simulink subsystem "Log"  (R2024b)
settings: Solver=VariableStepAuto  StartTime=0.0  StopTime=10.0  RelTol=1e-3
settings Model: Creator=Tong  LastModifiedBy=Tong

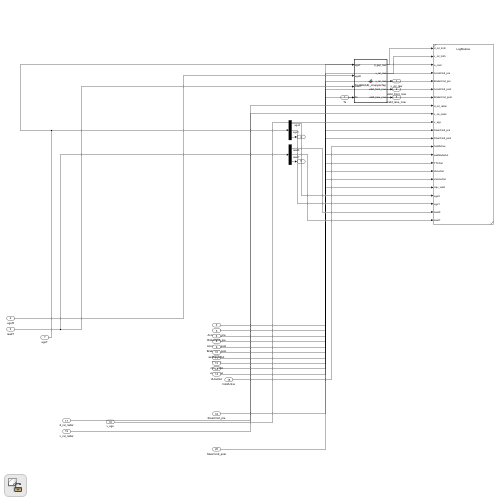
[thumbnail: Simulink's stored preview of the top-level diagram]
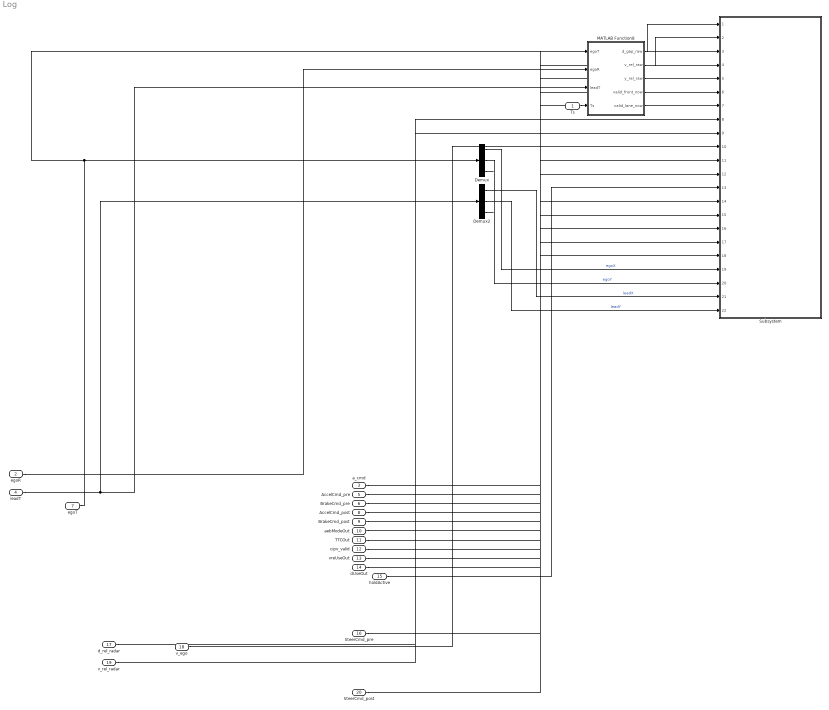
== system Log ==
  Ts : Inport
  egoR : Inport  Port=2
  a_cmd : Inport  Port=3
  leadT : Inport  Port=4
  AccelCmd_pre : Inport  Port=5
  BrakeCmd_pre : Inport  Port=6
  egoT : Inport  Port=7
  AccelCmd_post : Inport  Port=8
  BrakeCmd_post : Inport  Port=9
  aebModeOut : Inport  Port=10
  TTCOut : Inport  Port=11
  cipv_valid : Inport  Port=12
  vreUseOut : Inport  Port=13
  dUseOut : Inport  Port=14
  holdActive : Inport  Port=15
  SteerCmd_pre : Inport  Port=16
  d_rel_radar : Inport  Port=17
  v_ego : Inport  Port=18
  v_rel_radar : Inport  Port=19
  SteerCmd_post : Inport  Port=20
  Demux : Demux  Outputs=3
  Demux2 : Demux  Outputs=3
  MATLAB Function8 : MATLAB Function  TreatAsAtomicUnit=on
  Subsystem : Subsystem  ReferencedSubsystem=LogModule
  wires:
  MATLAB Function8/1(d_gap_raw) -> Subsystem/1
  leadT/1 -> Demux2/1, MATLAB Function8/3(leadT)
  Demux/3 -> ?
  MATLAB Function8/2(v_rel_raw) -> Subsystem/2
  dUseOut/1 -> Subsystem/16
  AccelCmd_post/1 -> Subsystem/6
  v_rel_radar/1 -> Subsystem/9
  Demux2/1 -> Subsystem/21  "leadX"
  SteerCmd_pre/1 -> Subsystem/11
  Demux2/2 -> Subsystem/22  "leadY"
  SteerCmd_post/1 -> Subsystem/12
  egoT/1 -> MATLAB Function8/1(egoT), Demux/1
  Demux/1 -> Subsystem/19  "egoX"
  aebModeOut/1 -> Subsystem/14
  Demux/2 -> Subsystem/20  "egoY"
  a_cmd/1 -> Subsystem/3
  MATLAB Function8/3(y_rel_raw) -> ?
  egoR/1 -> MATLAB Function8/2(egoR)
  Ts/1 -> MATLAB Function8/4(Ts)
  cipv_valid/1 -> Subsystem/18
  holdActive/1 -> Subsystem/13
  v_ego/1 -> Subsystem/10
  AccelCmd_pre/1 -> Subsystem/4
  BrakeCmd_post/1 -> Subsystem/7
  TTCOut/1 -> Subsystem/15
  vreUseOut/1 -> Subsystem/17
  Demux2/3 -> ?
  d_rel_radar/1 -> Subsystem/8
  BrakeCmd_pre/1 -> Subsystem/5
  MATLAB Function8/4(valid_front_now) -> ?
  MATLAB Function8/5(valid_lane_now) -> ?

== matlab function Log/MATLAB Function8 ==
  data: egoT input; d_gap_raw output; egoR input; leadT input; Ts input; v_rel_raw output; y_rel_raw output; valid_front_now output; valid_lane_now output
function [d_gap_raw, v_rel_raw, y_rel_raw, valid_front_now, valid_lane_now] = TruthRelUE_AnalysisTap(egoT, egoR, leadT, Ts)
%#codegen
% 并行分析函数（不参与控制）
% 输出原始分析量，不做 NO_TARGET_DIST 覆盖、不做 hold/coast 锁存
%
% 输出:
% d_gap_raw      : 原始前车gap距离(保险杠到保险杠, m, 可为0)
% v_rel_raw      : 原始相对速度(lead-ego, m/s)
% y_rel_raw      : 原始横向偏差(左正, m)
% valid_front_now: 当前帧仅“前方有效”判定
% valid_lane_now : 当前帧“前方+车道内”判定（无滞回）

%% 参数
Lego  = 4.7;
Llead = 4.7;
bumperComp = 0.5*(Lego + Llead);

LaneTh = 2.3;     % 分析判定可放宽
dMax   = 220;

% 速度滤波
fcV = 5; % Hz
alphaV = exp(-2*pi*fcV*Ts);

% 输出滤波
fcOut = 2; % Hz
alphaD = exp(-2*pi*fcOut*Ts);
alphaR = exp(-2*pi*fcOut*Ts);

% yaw估计
vHoldYaw   = 0.5;
maxYawRate = deg2rad(120);

%% 持久变量
persistent init egoPrev leadPrev egoVf leadVf yawF dFilt vFilt
if isempty(init)
    egoPrev = egoT(1:2)';
    leadPrev = leadT(1:2)';
    egoVf = [0;0];
    leadVf = [0;0];
    yawF = deg2rad(egoR(3)); % 初值
    dFilt = 0;
    vFilt = 0;
    init = true;
end

%% 1) 速度估计
egoNow  = egoT(1:2)';
leadNow = leadT(1:2)';

egoVraw  = (egoNow  - egoPrev) / Ts;
leadVraw = (leadNow - leadPrev) / Ts;
egoPrev  = egoNow;
leadPrev = leadNow;

egoVf  = alphaV*egoVf  + (1-alphaV)*egoVraw;
leadVf = alphaV*leadVf + (1-alphaV)*leadVraw;
vEgo = hypot(egoVf(1), egoVf(2));

%% 2) yaw估计（速度方向+限幅）
if vEgo >= vHoldYaw
    yawMeas = atan2(egoVf(2), egoVf(1));
    eYaw = wrapToPiLocal(yawMeas - yawF);
    maxStep = maxYawRate * Ts;
    if eYaw >  maxStep, eYaw =  maxStep; end
    if eYaw < -maxStep, eYaw = -maxStep; end
    yawF = wrapToPiLocal(yawF + eYaw);
end

c = cos(yawF); s = sin(yawF);

%% 3) 相对位移投影
dp = leadNow - egoNow;
dLong_center =  c*dp(1) + s*dp(2);
dLat         = -s*dp(1) + c*dp(2);

dGap = dLong_center - bumperComp;
if dGap < 0, dGap = 0; end

%% 4) 原始相对速度
vRel = c*(leadVf(1)-egoVf(1)) + s*(leadVf(2)-egoVf(2));

%% 5) 轻滤波（仅为画图平滑）
if dFilt == 0
    dFilt = dGap;
    vFilt = vRel;
else
    dFilt = alphaD*dFilt + (1-alphaD)*dGap;
    vFilt = alphaR*vFilt + (1-alphaR)*vRel;
end

d_gap_raw = dFilt;
v_rel_raw = vFilt;
y_rel_raw = dLat;

%% 6) 当前帧有效性（无滞回）
valid_front_now = (dGap > 0) && (dGap < dMax);
valid_lane_now  = valid_front_now && (abs(dLat) < LaneTh);

end

function y = wrapToPiLocal(x)
y = mod(x + pi, 2*pi) - pi;
end
